simulink model "PubIfDecisionLSM_MDL"  (R2020b)
settings: configuration reference "DspaceConfig" (kept outside this file)
PostLoadFcn:
  | if any(exist('dsrtsu_mdlpostloadfcn', 'file') ~= 0), dsrtsu_mdlpostloadfcn('Execute', bdroot); end
InitFcn:
  | , if any(exist('rtifpga_mdlclblib', 'file') ~= 0), rtifpga_mdlclblib('Init', bdroot); end,
  | , if any(exist('dsmpb_private', 'file') ~= 0), dsmpb_private('dsmpb_mdlclblib', 'Init', bdroot); end,
values from neighbouring files (symbols this model uses):
  P_LSM_ALC_Enable = 0.0    [LSM_Parameter.sldd]
  P_LSM_AwayEdge_offset = 0.1    [LSM_Parameter.sldd]
  P_LSM_CentValidErr = 1.0    [LSM_Parameter.sldd]
  P_LSM_DOP_C0_EN_Limit = 0.8    [LSM_Parameter.sldd]
  P_LSM_DOP_C0_out_Limit = 2.0    [LSM_Parameter.sldd]
  P_LSM_DOP_C1_EN_Limit : value not decoded    [LSM_Parameter.sldd]
  P_LSM_DOP_C1_out_Limit : value not decoded    [LSM_Parameter.sldd]
  P_LSM_DOP_C1AndC2_Lim_X : value not decoded    [LSM_Parameter.sldd]
  P_LSM_DOP_C2_EN_Limit : value not decoded    [LSM_Parameter.sldd]
  P_LSM_DOP_C2_out_Limit : value not decoded    [LSM_Parameter.sldd]
  P_LSM_DOP_In_Pre2Dop_Dis = 1.0    [LSM_Parameter.sldd]
  P_LSM_DOP_Out_Pre2Dop_Dis = 2.0    [LSM_Parameter.sldd]
  P_LSM_DOP_PreDis_X : value not decoded    [LSM_Parameter.sldd]
  P_LSM_DOP_PreDis_Y : value not decoded    [LSM_Parameter.sldd]
  P_LSM_DOPEnableSW = 1.0    [LSM_Parameter.sldd]
  P_LSM_DOPValid_CheckTime = 0.06    [LSM_Parameter.sldd]
  P_LSM_DoubleLine_Curr2Cent_Dislimit = 0.5    [LSM_Parameter.sldd]
  P_LSM_DoubleLine_Dop2Cent_Dislimit = 0.5    [LSM_Parameter.sldd]
  P_LSM_DoubleLine_DOPOut_C1 : value not decoded    [LSM_Parameter.sldd]
  P_LSM_DoubleLine_Pre2Cent_Dislimit = 1.0    [LSM_Parameter.sldd]
  P_LSM_Error_Limit = 0.5    [LSM_Parameter.sldd]
  P_LSM_IFV2CenterAxis = 0.0    [LSM_Parameter.sldd]
  P_LSM_IFV2RearAxis = 0.0    [LSM_Parameter.sldd]
  P_LSM_Line2Edge_limit = 0.5    [LSM_Parameter.sldd]
  P_LSM_Line_Error = 0.1    [LSM_Parameter.sldd]
  P_LSM_LineSTD_Limit = 0.15    [LSM_Parameter.sldd]
  P_LSM_NOH_Switch = 0.0    [LSM_Parameter.sldd]
  P_LSM_OTL_C0_Factor = 1.0    [LSM_Parameter.sldd]
  P_LSM_OTL_C1_Factor = 0.5    [LSM_Parameter.sldd]
  P_LSM_OTL_C2_Factor = 0.5    [LSM_Parameter.sldd]
  P_LSM_Pre2OnlyLineDis = 5.0    [LSM_Parameter.sldd]
  P_LSM_Pre_t = 0.0    [LSM_Parameter.sldd]
  P_LSM_SingleLine_Cent2Edge_Dislimit = 100.0    [LSM_Parameter.sldd]
  P_LSM_SingleLine_Curr2Cent_Dislimit = 0.2    [LSM_Parameter.sldd]
  P_LSM_SingleLine_Dop2Cent_Dislimit = 0.2    [LSM_Parameter.sldd]
  P_LSM_SingleLine_DOPOut_C1 : value not decoded    [LSM_Parameter.sldd]
  P_LSM_SingleLine_Pre2Cent_Dislimit = 0.5    [LSM_Parameter.sldd]
  P_LSM_TJALimitSpd = 60.0    [LSM_Parameter.sldd]
undefined symbols (not defined in the file or in its folder): P_lCS_IFV2CenterAxis, P_LCS_IFV2RearAxis, P_LSM_EntryEdge_offset, P_LSM_EntryLnChngEnSwitch, P_LSM_EntryVanishDis, P_LSM_LinetLostTime, P_LSM_LineWijCal_C12, P_LSM_LineWijCal_C13, P_LSM_MapValid_ErrorSwitch, P_LSM_PosLineLcFac, P_LSM_SpdLim_Stub_Spd, P_LSM_SpdLim_StubLength, P_LSM_SpdTurnAlarm
libraries: simulink x324, TrueDurationTime x11
(part 19 of 25)

== matlab function PubIfDecisionLSM_MDL/Subsystem1/TargetLineCalc_20ms2/TargetLineCalc/ESSLineCalc ==
  data: LeftLineTypeEn input boolean size=1; ESSLineValid output boolean size=1; RightLineTypeEn input boolean size=1; ESSSts input uint8 size=1; ESSStsK1 input uint8 size=1; LineConf input uint8 size=4; A3 input single size=4; A2 input single size=4; A1 input single size=4; A0 input single size=4; Range input single size=4; tLost input single size=4; EdgeValid input boolean size=2; EdgeA3 input single size=2; EdgeA2 input single size=2; EdgeA1 input single size=2; EdgeA0 input single size=2; dDeltaX input single size=1; dDeltaY input single size=1; CosOfPsi input single size=1; SinOfPsi input single size=1; LeftOffset_b input boolean size=1; RightOffset_b input boolean size=1; RoadWidth input single size=1; ESSDistLim input single size=1; ESSLineA3K1 input single size=1; ESSLineA2K1 input single size=1; ESSLineA1K1 input single size=1; ESSLineA0K1 input single size=1; ESSLeLineA3K1 input single size=1; ESSLineLA2K1 input single size=1; ESSLineLA1K1 input single size=1; ESSLineLA0K1 input single size=1; ESSLineRA3K1 input single size=1; ESSLineRA2K1 input single size=1; ESSLineRA1K1 input single size=1; ESSLineRA0K1 input single size=1; MoveIDK1 input int8 size=1; ESSLineC3 output single size=1; ESSLineC2 output single size=1; ESSLineC1 output single size=1; ESSLineC0 output single size=1; ESSRange output single size=1; ESSLeLineValid output boolean size=1; ESSLeLineC3 output single size=1; ESSLeLineC2 output single size=1; ESSLeLineC1 output single size=1; ESSLeLineC0 output single size=1; ESSLeRange output single size=1; ESSRiLineValid output boolean size=1; ESSRiLineC3 output single size=1; ESSRiLineC2 output single size=1; ESSRiLineC1 output single size=1; ESSRiLineC0 output single size=1; ESSRiRange output single size=1; MoveID output int8 size=1; Lock_bK1 input boolean size=1; Lock_b output boolean size=1
function [ESSLineValid,ESSLineC3,ESSLineC2,ESSLineC1,ESSLineC0,ESSRange,...
    ESSLeLineValid,ESSLeLineC3,ESSLeLineC2,ESSLeLineC1,ESSLeLineC0,ESSLeRange,...
    ESSRiLineValid,ESSRiLineC3,ESSRiLineC2,ESSRiLineC1,ESSRiLineC0,ESSRiRange,MoveID,Lock_b] = ...
    LineCalc(LeftLineTypeEn,RightLineTypeEn,ESSSts,ESSStsK1,LineConf,A3,A2,A1,A0,Range,tLost,...
    EdgeValid,EdgeA3,EdgeA2,EdgeA1,EdgeA0,...
    dDeltaX,dDeltaY,CosOfPsi,SinOfPsi,...
    LeftOffset_b,RightOffset_b,RoadWidth,ESSDistLim,...
    ESSLineA3K1,ESSLineA2K1,ESSLineA1K1,ESSLineA0K1,...
    ESSLeLineA3K1,ESSLineLA2K1,ESSLineLA1K1,ESSLineLA0K1,...
    ESSLineRA3K1,ESSLineRA2K1,ESSLineRA1K1,ESSLineRA0K1,...
    MoveIDK1,Lock_bK1)

ESSLineValid = false;
ESSLineC3 = single(0);
ESSLineC2 = single(0);
ESSLineC1 = single(0);
ESSLineC0 = single(0);
ESSRange = single(0);
ESSLeLineValid = false;
ESSLeLineC3 = single(0);
ESSLeLineC2 = single(0);
ESSLeLineC1 = single(0);
ESSLeLineC0 = single(0);
ESSLeRange = single(0);
ESSRiLineValid = false;
ESSRiLineC3 = single(0);
ESSRiLineC2 = single(0);
ESSRiLineC1 = single(0);
ESSRiLineC0 = single(0);
ESSRiRange = single(0);

MoveID = MoveIDK1;
Lock_b = Lock_bK1;

if (ESSSts==0)||(ESSSts==1)||(ESSSts==2)||(ESSSts==6)
    MoveID = int8(0);
    Lock_b = false;
%     if (LineConf(2)>0)&&(LineConf(3)>0)&&...
%             (Range(2)>ESSDistLim)&&(Range(3)>ESSDistLim)&&...
%             ((tLost(2)<0.15)||(tLost(3)<0.15))
%             ESSLineValid = true;
%             ESSLineA3 = 0.5*(A3(2) + A3(3));
%             ESSLineA2 = 0.5*(A2(2) + A2(3));
%             ESSLineA1 = 0.5*(A1(2) + A1(3));
%             ESSLineA0 = 0.5*(A0(2) + A0(3));
%             ESSLineRange = 0.5*(Range(2) + Range(3));
%     end
    if (LineConf(2)>0)&&(LineConf(1)>0)&&...
            (Range(2)>ESSDistLim)&&(Range(1)>ESSDistLim)&&...
            ((tLost(2)<0.15)||(tLost(1)<0.15))&&...
            (LeftLineTypeEn) && abs(A0(1)-A0(2))>3
        
        if EdgeValid(1)==true
            t = [0.1*ESSDistLim;0.3*ESSDistLim;0.6*ESSDistLim;ESSDistLim];
            t_EdgeDy = 0.25*EdgeA3(1)*t.^3 + 0.5*EdgeA2(1)*t.^2 + EdgeA1(1)*t + EdgeA0(1);
            t_LineLDy = A3(1)*t.^3 + A2(1)*t.^2 + A1(1)*t + A0(1);
            if min(t_EdgeDy - t_LineLDy)>0
                ESSLeLineValid = true;
                ESSLeLineC3 = 0.5*(A3(2) + A3(1));
                ESSLeLineC2 = 0.5*(A2(2) + A2(1));
                ESSLeLineC1 = 0.5*(A1(2) + A1(1));
                ESSLeLineC0 = 0.5*(A0(2) + A0(1));
                ESSLeRange = 0.5*(Range(2) + Range(1));
            end
        else
            ESSLeLineValid = true;
            ESSLeLineC3 = 0.5*(A3(2) + A3(1));
            ESSLeLineC2 = 0.5*(A2(2) + A2(1));
            ESSLeLineC1 = 0.5*(A1(2) + A1(1));
            ESSLeLineC0 = 0.5*(A0(2) + A0(1));
            ESSLeRange = 0.5*(Range(2) + Range(1));
        end
    end
    if (LineConf(4)>0)&&(LineConf(3)>0)&&...
            (Range(4)>ESSDistLim)&&(Range(3)>ESSDistLim)&&...
            ((tLost(4)<0.15)||(tLost(3)<0.15))&&...
            (RightLineTypeEn) && abs(A0(3)-A0(4))>3
        
        if EdgeValid(2)==true
            t = [0.1*ESSDistLim;0.3*ESSDistLim;0.6*ESSDistLim;ESSDistLim];
            t_EdgeDy = 0.25*EdgeA3(2)*t.^3 + 0.5*EdgeA2(2)*t.^2 + EdgeA1(2)*t + EdgeA0(2);
            t_LineLDy = A3(4)*t.^3 + A2(4)*t.^2 + A1(4)*t + A0(4);
            if min(t_LineLDy - t_EdgeDy)>0
                ESSRiLineValid = true;
                ESSRiLineC3 = 0.5*(A3(4) + A3(3));
                ESSRiLineC2 = 0.5*(A2(4) + A2(3));
                ESSRiLineC1 = 0.5*(A1(4) + A1(3));
                ESSRiLineC0 = 0.5*(A0(4) + A0(3));
                ESSRiRange = 0.5*(Range(4) + Range(3));
            end
        else
            ESSRiLineValid = true;
            ESSRiLineC3 = 0.5*(A3(4) + A3(3));
            ESSRiLineC2 = 0.5*(A2(4) + A2(3));
            ESSRiLineC1 = 0.5*(A1(4) + A1(3));
            ESSRiLineC0 = 0.5*(A0(4) + A0(3));
            ESSRiRange = 0.5*(Range(4) + Range(3));
        end
    end
elseif ESSSts==4
    if ESSStsK1~=4
        MoveID = MoveID - int8(1);
    end
    if LeftOffset_b
        MoveID = MoveID + int8(1);
    end
    if RightOffset_b
        MoveID = MoveID - int8(1);
    end
    if (MoveID>=1)||(MoveID<=-2)
        Error = true;
    else
        Error = false;
    end
    if Error==false
        if (LineConf(int8(2)+MoveID)>0)&&(LineConf(int8(3)+MoveID)>0)&&...
                (Range(int8(2)+MoveID)>0.8*ESSDistLim)&&(Range(int8(3)+MoveID)>0.8*ESSDistLim)
            Lock_b = false;
            ESSLineValid = true;
            ESSLineC3 = 0.5*(A3(int8(2)+MoveID) + A3(int8(3)+MoveID));
            ESSLineC2 = 0.5*(A2(int8(2)+MoveID) + A2(int8(3)+MoveID));
            ESSLineC1 = 0.5*(A1(int8(2)+MoveID) + A1(int8(3)+MoveID));
            ESSLineC0 = 0.5*(A0(int8(2)+MoveID) + A0(int8(3)+MoveID));
            ESSRange = 0.5*(Range(int8(2)+MoveID) + Range(int8(3)+MoveID));
            
            ESSLeLineValid = true;
            ESSLeLineC3 = 0.5*(A3(int8(2)+MoveID) + A3(int8(3)+MoveID));
            ESSLeLineC2 = 0.5*(A2(int8(2)+MoveID) + A2(int8(3)+MoveID));
            ESSLeLineC1 = 0.5*(A1(int8(2)+MoveID) + A1(int8(3)+MoveID));
            ESSLeLineC0 = 0.5*(A0(int8(2)+MoveID) + A0(int8(3)+MoveID));
            ESSLeRange = 0.5*(Range(int8(2)+MoveID) + Range(int8(3)+MoveID));
           elseif (LineConf(int8(2)+MoveID)>0)&&(Range(int8(2)+MoveID)>0.8*ESSDistLim)
            Lock_b = true;
            ESSLineValid = true;
            ESSLineA3 = A3(2+MoveID);
            ESSLineA2 = A2(2+MoveID);
            ESSLineA1 = A1(2+MoveID);
            ESSLineA0 = A0(2+MoveID)-0.5*RoadWidth*sqrt(1+A1(2+MoveID)*A1(2+MoveID));
            ESSLineRange = Range(2+MoveID);
            ESSLeLineValid = true;
            ESSLeLineA3 = ESSLineA3;
            ESSLeLineA2 = ESSLineA2;
            ESSLeLineA1 = ESSLineA1;
            ESSLeLineA0 = ESSLineA0;
            ESSLeRange =ESSLineRange;
%             SingleLineLost_b = true;
        elseif (LineConf(int8(3)+MoveID)>0)&&(Range(int8(3)+MoveID)>0.8*ESSDistLim)
            Lock_b = true;
            ESSLineValid = true;
            ESSLineA3 = A3(3+MoveID);
            ESSLineA2 = A2(3+MoveID);
            ESSLineA1 = A1(3+MoveID);
            ESSLineA0 = A0(3+MoveID)+0.5*RoadWidth*sqrt(1+A1(3+MoveID)*A1(3+MoveID));
            ESSLineRange = Range(3+MoveID);
            ESSLeLineValid = true;
            ESSLeLineA3 = ESSLineA3;
            ESSLeLineA2 = ESSLineA2;
            ESSLeLineA1 = ESSLineA1;
            ESSLeLineA0 = ESSLineA0;
            ESSLeRange =ESSLineRange;
%             SingleLineLost_b = true; 
%         else
%             Lock_b = true;
%             MoveID = int8(0);
%             if ESSStsK1~=4
%                 xi = [0;10;20;40];
%                 yi = ESSLineLA3K1*xi.^3 + ESSLineLA2K1*xi.^2 + ESSLineLA1K1*xi + ESSLineLA0K1;
%                 t_dx = xi-dDeltaX;
%                 t_dy = yi-dDeltaY;
%                 TmpX = t_dx*CosOfPsi+t_dy*SinOfPsi;
%                 TmpY = -t_dx*SinOfPsi+t_dy*CosOfPsi;
%                 [ESSLineC3,ESSLineC2,ESSLineC1,ESSLineC0] = pl(TmpX,TmpY);
%                 ESSLineValid = true;
%             else
%                 xi = [0;10;20;40];
%                 yi = ESSLineA3K1*xi.^3 + ESSLineA2K1*xi.^2 + ESSLineA1K1*xi + ESSLineA0K1;
%                 t_dx = xi-dDeltaX;
%                 t_dy = yi-dDeltaY;
%                 TmpX = t_dx*CosOfPsi+t_dy*SinOfPsi;
%                 TmpY = -t_dx*SinOfPsi+t_dy*CosOfPsi;
%                 [ESSLineC3,ESSLineC2,ESSLineC1,ESSLineC0] = pl(TmpX,TmpY);
%                 ESSLineValid = true;
            end
        end
    end
elseif ESSSts==5
    if ESSStsK1~=5
        MoveID = MoveID + int8(1);
    end
    if LeftOffset_b
        MoveID = MoveID + int8(1);
    end
    if RightOffset_b
        MoveID = MoveID - int8(1);
    end
    if (MoveID>=2)||(MoveID<=-1)
        Error = true;
    else
        Error = false;
    end
    if Error==false
        if (Lock_b==false)&&...
                (LineConf(int8(2)+MoveID)>0)&&(LineConf(int8(3)+MoveID)>0)&&...
                (Range(int8(2)+MoveID)>0.8*ESSDistLim)&&(Range(int8(3)+MoveID)>0.8*ESSDistLim)
            
            ESSLineValid = true;
            ESSLineC3 = 0.5*(A3(int8(2)+MoveID) + A3(int8(3)+MoveID));
            ESSLineC2 = 0.5*(A2(int8(2)+MoveID) + A2(int8(3)+MoveID));
            ESSLineC1 = 0.5*(A1(int8(2)+MoveID) + A1(int8(3)+MoveID));
            ESSLineC0 = 0.5*(A0(int8(2)+MoveID) + A0(int8(3)+MoveID));
            ESSRange = 0.5*(Range(int8(2)+MoveID) + Range(int8(3)+MoveID));
            
            ESSRiLineValid = true;
            ESSRiLineC3 = 0.5*(A3(int8(2)+MoveID) + A3(int8(3)+MoveID));
            ESSRiLineC2 = 0.5*(A2(int8(2)+MoveID) + A2(int8(3)+MoveID));
            ESSRiLineC1 = 0.5*(A1(int8(2)+MoveID) + A1(int8(3)+MoveID));
            ESSRiLineC0 = 0.5*(A0(int8(2)+MoveID) + A0(int8(3)+MoveID));
            ESSRiRange = 0.5*(Range(int8(2)+MoveID) + Range(int8(3)+MoveID));
        else
            Lock_b = true;
            MoveID = int8(0);
            if ESSStsK1~=5
                xi = [0;10;20;40];
                yi = ESSLineRA3K1*xi.^3 + ESSLineRA2K1*xi.^2 + ESSLineRA1K1*xi + ESSLineRA0K1;
                t_dx = xi-dDeltaX;
                t_dy = yi-dDeltaY;
                TmpX = t_dx*CosOfPsi+t_dy*SinOfPsi;
                TmpY = -t_dx*SinOfPsi+t_dy*CosOfPsi;
                [ESSLineC3,ESSLineC2,ESSLineC1,ESSLineC0] = pl(TmpX,TmpY);
                ESSLineValid = true;
            else
                xi = [0;10;20;40];
                yi = ESSLineA3K1*xi.^3 + ESSLineA2K1*xi.^2 + ESSLineA1K1*xi + ESSLineA0K1;
                t_dx = xi-dDeltaX;
                t_dy = yi-dDeltaY;
                TmpX = t_dx*CosOfPsi+t_dy*SinOfPsi;
                TmpY = -t_dx*SinOfPsi+t_dy*CosOfPsi;
                [ESSLineC3,ESSLineC2,ESSLineC1,ESSLineC0] = pl(TmpX,TmpY);
                ESSLineValid = true;
            end
        end
    end 
end
end

== matlab function PubIfDecisionLSM_MDL/Subsystem1/TargetLineCalc_20ms2/TargetLineCalc/ESSLineCalc1 ==
  data: LeftLineTypeEn input boolean; ESSLineValid output boolean; RightLineTypeEn input boolean; ESSSts input uint8; ESSStsK1 input uint8; LineConf input uint8; A3 input single; A2 input single; A1 input single; A0 input single; Range input single; tLost input single; EdgeValid input boolean; EdgeA3 input single; EdgeA2 input single; EdgeA1 input single; EdgeA0 input single; LeftOffset_b input boolean; RightOffset_b input boolean; RoadWidth input single; ESSDistLim input single; MoveIDK1 input int8; ESSLineA3 output single; ESSLineA2 output single; ESSLineA1 output single; ESSLineA0 output single; ESSRange output single; ESSLeLineValid output boolean; ESSLeLineA3 output single; ESSLeLineA2 output single; ESSLeLineA1 output single; ESSLeLineA0 output single; ESSLeRange output single; ESSRiLineValid output boolean; ESSRiLineA3 output single; ESSRiLineA2 output single; ESSRiLineA1 output single; ESSRiLineA0 output single; ESSRiRange output single; MoveID output int8; Lock_bK1 input boolean; Lock_b output boolean
function [ESSLineValid,ESSLineA3,ESSLineA2,ESSLineA1,ESSLineA0,ESSRange,...
    ESSLeLineValid,ESSLeLineA3,ESSLeLineA2,ESSLeLineA1,ESSLeLineA0,ESSLeRange,...
    ESSRiLineValid,ESSRiLineA3,ESSRiLineA2,ESSRiLineA1,ESSRiLineA0,ESSRiRange,MoveID,Lock_b] = ...
    LineCalc(LeftLineTypeEn,RightLineTypeEn,ESSSts,ESSStsK1,LineConf,A3,A2,A1,A0,Range,tLost,...
    EdgeValid,EdgeA3,EdgeA2,EdgeA1,EdgeA0,...
    LeftOffset_b,RightOffset_b,RoadWidth,ESSDistLim,...
    MoveIDK1,Lock_bK1)

ESSLineValid = false;
ESSLineA3 = single(0);
ESSLineA2 = single(0);
ESSLineA1 = single(0);
ESSLineA0 = single(0);
ESSRange = single(0);
ESSLeLineValid = false;
ESSLeLineA3 = single(0);
ESSLeLineA2 = single(0);
ESSLeLineA1 = single(0);
ESSLeLineA0 = single(0);
ESSLeRange = single(0);
ESSRiLineValid = false;
ESSRiLineA3 = single(0);
ESSRiLineA2 = single(0);
ESSRiLineA1 = single(0);
ESSRiLineA0 = single(0);
ESSRiRange = single(0);
% SingleLineLost_b = false;
% DoubleLineLost_b = false;
MoveID = MoveIDK1;
Lock_b = Lock_bK1;

if (ESSSts==0)||(ESSSts==1)||(ESSSts==2)||(ESSSts==6)
    MoveID = int8(0);
    Lock_b = false;             %add
%         if (LineConf(2)>0)&&(LineConf(3)>0)&&...
%                 (Range(2)>ESSDistLim)&&(Range(3)>ESSDistLim)&&...
%                 ((tLost(2)<0.15)||(tLost(3)<0.15))
%                 ESSLineValid = true;
%                 ESSLineA3 = 0.5*(A3(2) + A3(3));
%                 ESSLineA2 = 0.5*(A2(2) + A2(3));
%                 ESSLineA1 = 0.5*(A1(2) + A1(3));
%                 ESSLineA0 = 0.5*(A0(2) + A0(3));
%                 ESSLineRange = 0.5*(Range(2) + Range(3));
%         end
    if (LineConf(2)>0)&&(LineConf(1)>0)&&...
            (Range(2)>ESSDistLim)&&(Range(1)>ESSDistLim)&&...
            ((tLost(2)<0.15)||(tLost(1)<0.15))&&...
            (LeftLineTypeEn)
        
        if EdgeValid(1)==true
            t = [0.1*ESSDistLim;0.3*ESSDistLim;0.6*ESSDistLim;ESSDistLim];
            t_EdgeDy = 0.25*EdgeA3(1)*t.^3 + 0.5*EdgeA2(1)*t.^2 + EdgeA1(1)*t + EdgeA0(1);
            t_LineLDy = A3(1)*t.^3 + A2(1)*t.^2 + A1(1)*t + A0(1);
            if min(t_EdgeDy - t_LineLDy)>0
                ESSLeLineValid = true;
                ESSLeLineA3 = 0.5*(A3(2) + A3(1));
                ESSLeLineA2 = 0.5*(A2(2) + A2(1));
                ESSLeLineA1 = 0.5*(A1(2) + A1(1));
                ESSLeLineA0 = 0.5*(A0(2) + A0(1));
                ESSLeRange = 0.5*(Range(2) + Range(1));
            end
        else
            ESSLeLineValid = true;
            ESSLeLineA3 = 0.5*(A3(2) + A3(1));
            ESSLeLineA2 = 0.5*(A2(2) + A2(1));
            ESSLeLineA1 = 0.5*(A1(2) + A1(1));
            ESSLeLineA0 = 0.5*(A0(2) + A0(1));
            ESSLeRange = 0.5*(Range(2) + Range(1));
        end
    end
    if (LineConf(4)>0)&&(LineConf(3)>0)&&...
            (Range(4)>ESSDistLim)&&(Range(3)>ESSDistLim)&&...
            ((tLost(4)<0.15)||(tLost(3)<0.15))&&...
            (RightLineTypeEn)
        
        if EdgeValid(2)==true
            t = [0.1*ESSDistLim;0.3*ESSDistLim;0.6*ESSDistLim;ESSDistLim];
            t_EdgeDy = 0.25*EdgeA3(2)*t.^3 + 0.5*EdgeA2(2)*t.^2 + EdgeA1(2)*t + EdgeA0(2);
            t_LineLDy = A3(4)*t.^3 + A2(4)*t.^2 + A1(4)*t + A0(4);
            if min(t_LineLDy - t_EdgeDy)>0
                ESSRiLineValid = true;
                ESSRiLineA3 = 0.5*(A3(4) + A3(3));
                ESSRiLineA2 = 0.5*(A2(4) + A2(3));
                ESSRiLineA1 = 0.5*(A1(4) + A1(3));
                ESSRiLineA0 = 0.5*(A0(4) + A0(3));
                ESSRiRange = 0.5*(Range(4) + Range(3));
            end
        else
            ESSRiLineValid = true;
            ESSRiLineA3 = 0.5*(A3(4) + A3(3));
            ESSRiLineA2 = 0.5*(A2(4) + A2(3));
            ESSRiLineA1 = 0.5*(A1(4) + A1(3));
            ESSRiLineA0 = 0.5*(A0(4) + A0(3));
            ESSRiRange = 0.5*(Range(4) + Range(3));
        end
    end
elseif ESSSts==4
    if ESSStsK1~=4
        MoveID = MoveID - int8(1);
    end
    if LeftOffset_b
        MoveID = MoveID + int8(1);
    end
    if RightOffset_b
        MoveID = MoveID - int8(1);
    end
    if (MoveID>=1)||(MoveID<=-2)
        Error = true;
    else
        Error = false;
    end
    if Error==false
        if  (LineConf(int8(2)+MoveID)>0)&&(LineConf(int8(3)+MoveID)>0)&&...
                (Range(int8(2)+MoveID)>0.8*ESSDistLim)&&(Range(int8(3)+MoveID)>0.8*ESSDistLim)
%                 &&(abs(A0(int8(2)+MoveID)-A0(int8(3)+MoveID))>=0.8*RoadWidth)...     %add
%                 &&(VisLineConf(int8(2)+MoveID)>0)&&(VisLineConf(int8(3)+MoveID)>0)   %add
            Lock_b = false;
            ESSLineValid = true;
            ESSLineA3 = 0.5*(A3(int8(2)+MoveID) + A3(int8(3)+MoveID));
            ESSLineA2 = 0.5*(A2(int8(2)+MoveID) + A2(int8(3)+MoveID));
            ESSLineA1 = 0.5*(A1(int8(2)+MoveID) + A1(int8(3)+MoveID));
            ESSLineA0 = 0.5*(A0(int8(2)+MoveID) + A0(int8(3)+MoveID));
            ESSRange = 0.5*(Range(int8(2)+MoveID) + Range(int8(3)+MoveID));
            
            ESSLeLineValid = true;
            ESSLeLineA3 = 0.5*(A3(int8(2)+MoveID) + A3(int8(3)+MoveID));
            ESSLeLineA2 = 0.5*(A2(int8(2)+MoveID) + A2(int8(3)+MoveID));
            ESSLeLineA1 = 0.5*(A1(int8(2)+MoveID) + A1(int8(3)+MoveID));
            ESSLeLineA0 = 0.5*(A0(int8(2)+MoveID) + A0(int8(3)+MoveID));
            ESSLeRange = 0.5*(Range(int8(2)+MoveID) + Range(int8(3)+MoveID));
        elseif (LineConf(int8(2)+MoveID)>0)&&(Range(int8(2)+MoveID)>0.8*ESSDistLim)
            Lock_b = true;
            ESSLineValid = true;
            ESSLineA3 = A3(2+MoveID);
            ESSLineA2 = A2(2+MoveID);
            ESSLineA1 = A1(2+MoveID);
            ESSLineA0 = A0(2+MoveID)-0.5*RoadWidth*sqrt(1+A1(2+MoveID)*A1(2+MoveID));
            ESSRange = Range(2+MoveID);
            ESSLeLineValid = true;
            ESSLeLineA3 = ESSLineA3;
            ESSLeLineA2 = ESSLineA2;
            ESSLeLineA1 = ESSLineA1;
            ESSLeLineA0 = ESSLineA0;
            ESSLeRange =ESSRange;
        elseif (LineConf(int8(3)+MoveID)>0)&&(Range(int8(3)+MoveID)>0.8*ESSDistLim)
            Lock_b = true;
            ESSLineValid = true;
            ESSLineA3 = A3(3+MoveID);
            ESSLineA2 = A2(3+MoveID);
            ESSLineA1 = A1(3+MoveID);
            ESSLineA0 = A0(3+MoveID)+0.5*RoadWidth*sqrt(1+A1(3+MoveID)*A1(3+MoveID));
            ESSRange = Range(3+MoveID);
            ESSLeLineValid = true;
            ESSLeLineA3 = ESSLineA3;
            ESSLeLineA2 = ESSLineA2;
            ESSLeLineA1 = ESSLineA1;
            ESSLeLineA0 = ESSLineA0;
            ESSLeRange =ESSRange;
            %             MoveID = int8(0);
%             if ESSStsK1~=4
%                 xi = [0;10;20;40];
%                 yi = ESSLineLA3K1*xi.^3 + ESSLineLA2K1*xi.^2 + ESSLineLA1K1*xi + ESSLineLA0K1;
%                 t_dx = xi-dDeltaX;
%                 t_dy = yi-dDeltaY;
%                 TmpX = t_dx*CosOfPsi+t_dy*SinOfPsi;
%                 TmpY = -t_dx*SinOfPsi+t_dy*CosOfPsi;
%                 [ESSLineLA3,ESSLineLA2,ESSLineLA1,ESSLineLA0] = pl(TmpX,TmpY);
%                 ESSLineLValid = true;
%                 [ESSLineA3,ESSLineA2,ESSLineA1,ESSLineA0] = pl(TmpX,TmpY);
%                 ESSLineValid = true;
%             else
%                 xi = [0;10;20;40];
%                 yi = ESSLineLA3K1*xi.^3 + ESSLineLA2K1*xi.^2 + ESSLineLA1K1*xi + ESSLineLA0K1;
%                 t_dx = xi-dDeltaX;
%                 t_dy = yi-dDeltaY;
%                 TmpX = t_dx*CosOfPsi+t_dy*SinOfPsi;
%                 TmpY = -t_dx*SinOfPsi+t_dy*CosOfPsi;
%                 [ESSLineLA3,ESSLineLA2,ESSLineLA1,ESSLineLA0] = pl(TmpX,TmpY);
%                 ESSLineLValid = true;
%                 [ESSLineA3,ESSLineA2,ESSLineA1,ESSLineA0] = pl(TmpX,TmpY);
%                 ESSLineValid = true;
%             end
        end
    end
elseif ESSSts==5
    if ESSStsK1~=5
        MoveID = MoveID + int8(1);
    end
    if LeftOffset_b
        MoveID = MoveID + int8(1);
    end
    if RightOffset_b
        MoveID = MoveID - int8(1);
    end
    if (MoveID>=2)||(MoveID<=-1)
        Error = true;
    else
        Error = false;
    end
    if Error==false
        if (LineConf(int8(2)+MoveID)>0)&&(LineConf(int8(3)+MoveID)>0)&&...
                (Range(int8(2)+MoveID)>0.8*ESSDistLim)&&(Range(int8(3)+MoveID)>0.8*ESSDistLim)
%                 &&(abs(A0(int8(2)+MoveID)-A0(int8(3)+MoveID))>=0.8*RoadWidth)...             %add
%                 &&(VisLineConf(int8(2)+MoveID)>0)&&(VisLineConf(int8(3)+MoveID)>0)           %add
            Lock_b = false;
            ESSLineValid = true;
            ESSLineA3 = 0.5*(A3(int8(2)+MoveID) + A3(int8(3)+MoveID));
            ESSLineA2 = 0.5*(A2(int8(2)+MoveID) + A2(int8(3)+MoveID));
            ESSLineA1 = 0.5*(A1(int8(2)+MoveID) + A1(int8(3)+MoveID));
            ESSLineA0 = 0.5*(A0(int8(2)+MoveID) + A0(int8(3)+MoveID));
            ESSRange = 0.5*(Range(int8(2)+MoveID) + Range(int8(3)+MoveID));
            
            ESSRiLineValid = true;
            ESSRiLineA3 = 0.5*(A3(int8(2)+MoveID) + A3(int8(3)+MoveID));
            ESSRiLineA2 = 0.5*(A2(int8(2)+MoveID) + A2(int8(3)+MoveID));
            ESSRiLineA1 = 0.5*(A1(int8(2)+MoveID) + A1(int8(3)+MoveID));
            ESSRiLineA0 = 0.5*(A0(int8(2)+MoveID) + A0(int8(3)+MoveID));
            ESSRiRange = 0.5*(Range(int8(2)+MoveID) + Range(int8(3)+MoveID));
        elseif (LineConf(int8(2)+MoveID)>0)&&(Range(int8(2)+MoveID)>0.8*ESSDistLim)
            Lock_b = true;
            ESSLineValid = true;
            ESSLineA3 = A3(2+MoveID);
            ESSLineA2 = A2(2+MoveID);
            ESSLineA1 = A1(2+MoveID);
            ESSLineA0 = A0(2+MoveID)-0.5*RoadWidth*sqrt(1+A1(2+MoveID)*A1(2+MoveID));
            ESSRange = Range(2+MoveID);
            ESSRiLineValid = true;
            ESSRiLineA3 = ESSLineA3;
            ESSRiLineA2 = ESSLineA2;
            ESSRiLineA1 = ESSLineA1;
            ESSRiLineA0 = ESSLineA0;
            ESSRiRange =ESSRange;
        elseif (LineConf(int8(3)+MoveID)>0)&&(Range(int8(3)+MoveID)>0.8*ESSDistLim)
            Lock_b = true;
            ESSLineValid = true;
            ESSLineA3 = A3(3+MoveID);
            ESSLineA2 = A2(3+MoveID);
            ESSLineA1 = A1(3+MoveID);
            ESSLineA0 = A0(3+MoveID)+0.5*RoadWidth*sqrt(1+A1(3+MoveID)*A1(3+MoveID));
            ESSRange = Range(3+MoveID);
            ESSRiLineValid = true;
            ESSRiLineA3 = ESSLineA3;
            ESSRiLineA2 = ESSLineA2;
            ESSRiLineA1 = ESSLineA1;
            ESSRiLineA0 = ESSLineA0;
            ESSRiRange =ESSRange;
            %             MoveID = int8(0);
%             if ESSStsK1~=5
%                 xi = [0;10;20;40];
%                 yi = ESSLineRA3K1*xi.^3 + ESSLineRA2K1*xi.^2 + ESSLineRA1K1*xi + ESSLineRA0K1;
%                 t_dx = xi-dDeltaX;
%                 t_dy = yi-dDeltaY;
%                 TmpX = t_dx*CosOfPsi+t_dy*SinOfPsi;
%                 TmpY = -t_dx*SinOfPsi+t_dy*CosOfPsi;
%                 [ESSLineA3,ESSLineA2,ESSLineA1,ESSLineA0] = pl(TmpX,TmpY);
%                 ESSLineValid = true;
%                 [ESSLineRA3,ESSLineRA2,ESSLineRA1,ESSLineRA0] = pl(TmpX,TmpY);
%                 ESSLineRValid = true;
%             else
%                 xi = [0;10;20;40];
%                 yi = ESSLineRA3K1*xi.^3 + ESSLineRA2K1*xi.^2 + ESSLineRA1K1*xi + ESSLineRA0K1;
%                 t_dx = xi-dDeltaX;
%                 t_dy = yi-dDeltaY;
%                 TmpX = t_dx*CosOfPsi+t_dy*SinOfPsi;
%                 TmpY = -t_dx*SinOfPsi+t_dy*CosOfPsi;
%                 [ESSLineRA3,ESSLineRA2,ESSLineRA1,ESSLineRA0] = pl(TmpX,TmpY);
%                 ESSLineRValid = true;
%                 [ESSLineA3,ESSLineA2,ESSLineA1,ESSLineA0] = pl(TmpX,TmpY);
%                 ESSLineValid = true;
%             end
        end
    end
end
